simulink model "PassStCalib"  (R2024b)
settings: Solver=FixedStepDiscrete  StartTime=0.0  StopTime=10.0  FixedStep=0.01  RelTol=1e-3
model workspace (MAT data in the model file):
  KeSMSwAcsEntryPassStBkReclnUpwdDnwdPosMax_Val : Simulink.Parameter (value not decoded)
  KeSMSwAcsEntryPassStBkReclnUpwdDnwdPosMin_Val : Simulink.Parameter (value not decoded)
  KeSMSwAcsEntryPassStBkReclnUpwdDnwdPos_Val : Simulink.Parameter (value not decoded)
  KeSMSwAcsEntryPassStFrwdBkwdPosMax_Val : Simulink.Parameter (value not decoded)
  KeSMSwAcsEntryPassStFrwdBkwdPosMin_Val : Simulink.Parameter (value not decoded)
  KeSMSwAcsEntryPassStFrwdBkwdPos_Val : Simulink.Parameter (value not decoded)
  KeSMSwAcsMd56PassStBkReclnUpwdDnwdPosMax_Val : Simulink.Parameter (value not decoded)
  KeSMSwAcsMd56PassStBkReclnUpwdDnwdPosMin_Val : Simulink.Parameter (value not decoded)
  KeSMSwAcsMd56PassStBkReclnUpwdDnwdPos_Val : Simulink.Parameter (value not decoded)
  KeSMSwAcsMd56PassStFrwdBkwdPosMax_Val : Simulink.Parameter (value not decoded)
  KeSMSwAcsMd56PassStFrwdBkwdPosMin_Val : Simulink.Parameter (value not decoded)
  KeSMSwAcsMd56PassStFrwdBkwdPos_Val : Simulink.Parameter (value not decoded)
  KeSMSwRevRMDPassStBkReclnUpwdDnwdPosMax_Val : Simulink.Parameter (value not decoded)
  KeSMSwRevRMDPassStBkReclnUpwdDnwdPosMin_Val : Simulink.Parameter (value not decoded)
  KeSMSwRevRMDPassStBkReclnUpwdDnwdPos_Val : Simulink.Parameter (value not decoded)
  KeSMSwRevRMDPassStFrwdBkwdPosMax_Val : Simulink.Parameter (value not decoded)
  KeSMSwRevRMDPassStFrwdBkwdPosMin_Val : Simulink.Parameter (value not decoded)
  KeSMSwRevRMDPassStFrwdBkwdPos_Val : Simulink.Parameter (value not decoded)
symbols that are objects in the model workspace (value not decoded): KeSMSwAcsEntryPassStBkReclnUpwdDnwdPos_Val, KeSMSwAcsEntryPassStBkReclnUpwdDnwdPosMax_Val, KeSMSwAcsEntryPassStBkReclnUpwdDnwdPosMin_Val, KeSMSwAcsEntryPassStFrwdBkwdPos_Val, KeSMSwAcsEntryPassStFrwdBkwdPosMax_Val, KeSMSwAcsEntryPassStFrwdBkwdPosMin_Val, KeSMSwAcsMd56PassStBkReclnUpwdDnwdPos_Val, KeSMSwAcsMd56PassStBkReclnUpwdDnwdPosMax_Val, KeSMSwAcsMd56PassStBkReclnUpwdDnwdPosMin_Val, KeSMSwAcsMd56PassStFrwdBkwdPos_Val, KeSMSwAcsMd56PassStFrwdBkwdPosMax_Val, KeSMSwAcsMd56PassStFrwdBkwdPosMin_Val, KeSMSwRevRMDPassStBkReclnUpwdDnwdPos_Val, KeSMSwRevRMDPassStBkReclnUpwdDnwdPosMax_Val, KeSMSwRevRMDPassStBkReclnUpwdDnwdPosMin_Val, KeSMSwRevRMDPassStFrwdBkwdPos_Val, KeSMSwRevRMDPassStFrwdBkwdPosMax_Val, KeSMSwRevRMDPassStFrwdBkwdPosMin_Val
undefined symbols (not defined in the file or in its folder): KeSMSuSecRwStVIPFtrstRefAngle_Val, KeSMSw6sAcsEntryPassStFtUpwdDnwdPos_Val, KeSMSw6sAcsEntryPassStFtUpwdDnwdPosMiax_Val, KeSMSw6sAcsEntryPassStFtUpwdDnwdPosMin_Val, KeSMSw6sAcsExtPassStFtUpwdDnwdPos_Val, KeSMSw6sAcsExtPassStFtUpwdDnwdPosMax_Val, KeSMSw6sAcsExtPassStFtUpwdDnwdPosMin_Val, KeSMSw6sRecoveryPassStStFtUpwdDnwdPos_Val, KeSMSw6sRecoveryPassStStFtUpwdDnwdPosMax_Val, KeSMSw6sRecoveryPassStStFtUpwdDnwdPosMin_Val, KeSMSw6SVIPMdPassStBkReclnUpwdDnwdPosPos_Val, KeSMSw6SVIPMdPassStBkReclnUpwdDnwdPosPosMax_Val, KeSMSw6SVIPMdPassStBkReclnUpwdDnwdPosPosMin_Val, KeSMSw6SVIPMdPassStFrwdBkwdPos2_Val, KeSMSw6SVIPMdPassStFrwdBkwdPosMax2_Val, KeSMSw6SVIPMdPassStFrwdBkwdPosMin2_Val, KeSMSw6SVIPMdPassStFrwdBkwdPosPos_Val, KeSMSw6SVIPMdPassStFrwdBkwdPosPosMax_Val, KeSMSw6SVIPMdPassStFrwdBkwdPosPosMin_Val, KeSMSwAcsEntryPassStFtUpwdDnwdPos_Val, KeSMSwAcsEntryPassStFtUpwdDnwdPosMiax_Val, KeSMSwAcsEntryPassStFtUpwdDnwdPosMin_Val, KeSMSwAcsExtPassStFtUpwdDnwdPos_Val, KeSMSwAcsExtPassStFtUpwdDnwdPosMax_Val, KeSMSwAcsExtPassStFtUpwdDnwdPosMin_Val, KeSMSwAcsMd30PassStBkReclnUpwdDnwdPos1_Val, KeSMSwAcsMd30PassStBkReclnUpwdDnwdPos1Max_Val, KeSMSwAcsMd30PassStBkReclnUpwdDnwdPos1Min_Val, KeSMSwAcsMd30PassStBkReclnUpwdDnwdPos_Val, KeSMSwAcsMd30PassStBkReclnUpwdDnwdPosMax_Val, KeSMSwAcsMd30PassStBkReclnUpwdDnwdPosMin_Val, KeSMSwAcsMd30PassStFldUpwdDnwdPos1_Val, KeSMSwAcsMd30PassStFldUpwdDnwdPos1Max_Val, KeSMSwAcsMd30PassStFldUpwdDnwdPos1Min_Val, KeSMSwAcsMd30PassStFldUpwdDnwdPos_Val, KeSMSwAcsMd30PassStFldUpwdDnwdPosMax_Val, KeSMSwAcsMd30PassStFldUpwdDnwdPosMin_Val, KeSMSwAcsMd30PassStFrwdBkwdPos1_Val, KeSMSwAcsMd30PassStFrwdBkwdPos1Max_Val, KeSMSwAcsMd30PassStFrwdBkwdPos1Min_Val, KeSMSwAcsMd30PassStFrwdBkwdPos_Val, KeSMSwAcsMd30PassStFrwdBkwdPosMax_Val, KeSMSwAcsMd30PassStFrwdBkwdPosMin_Val, KeSMSwAcsMd31PassStBkReclnUpwdDnwdPos1_Val, KeSMSwAcsMd31PassStBkReclnUpwdDnwdPos1Max_Val, KeSMSwAcsMd31PassStBkReclnUpwdDnwdPos1Min_Val, KeSMSwAcsMd31PassStBkReclnUpwdDnwdPos_Val, KeSMSwAcsMd31PassStBkReclnUpwdDnwdPosMax_Val, KeSMSwAcsMd31PassStBkReclnUpwdDnwdPosMin_Val, KeSMSwAcsMd31PassStFldUpwdDnwdPos_Val, KeSMSwAcsMd31PassStFldUpwdDnwdPosMax_Val, KeSMSwAcsMd31PassStFldUpwdDnwdPosMin_Val, KeSMSwAcsMd31PassStFrwdBkwdPos1_Val, KeSMSwAcsMd31PassStFrwdBkwdPos1Max_Val, KeSMSwAcsMd31PassStFrwdBkwdPos1Min_Val, KeSMSwAcsMd31PassStFrwdBkwdPos_Val, KeSMSwAcsMd31PassStFrwdBkwdPosMax_Val, KeSMSwAcsMd31PassStFrwdBkwdPosMin_Val, KeSMSwAcsMd57PassStBkReclnUpwdDnwdPosPos_Val, KeSMSwAcsMd57PassStBkReclnUpwdDnwdPosPosMax_Val ... (+34)
libraries: TrgtPosSelcLib x20
(part 3 of 3)

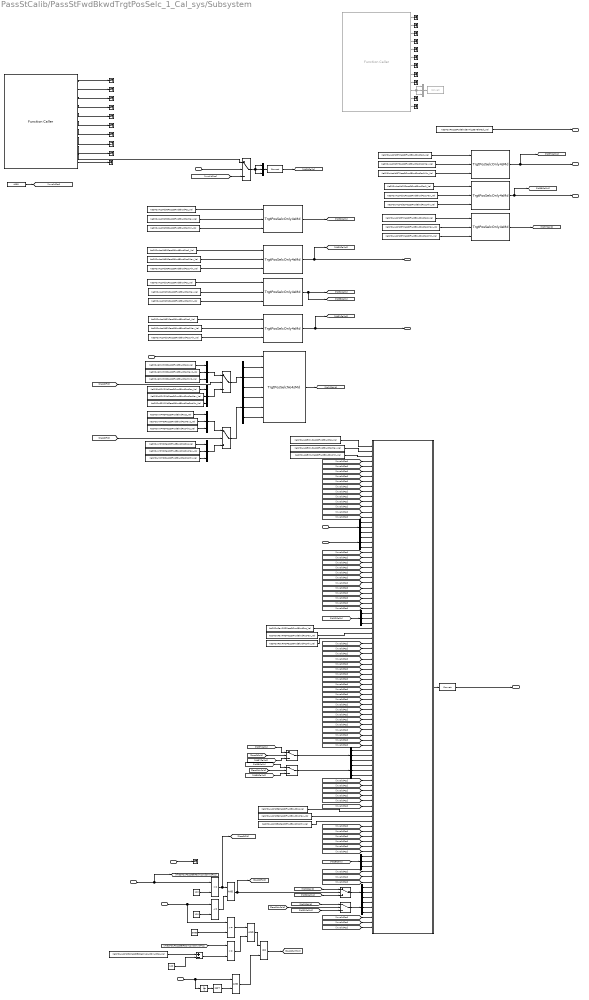
== system PassStCalib/PassStFwdBkwdTrgtPosSelc_1_Cal_sys/Subsystem ==
  note: 副驾折叠判断条件更改
  note: Delete block
  IfVeSMSbSecRwRtStCshnFrntUpwdDnwdMovConfig_Val_read : Inport
  Md30BkStgDone_Val_read : Inport  Port=2
  Md31BkStgDone_Val_read : Inport  Port=3
  StNumFlg_Is6s_read : Inport  Port=4
  IfVeSMSuPassStBkReclnUpwdDnwdPos_Val_read : Inport  Port=5
  IfVeSMSuPassStFldUpwdDnwdPos_Val_read : Inport  Port=6
  Md61PassStFwdBkwdTrgtPosCalib_TrgtPosArray_read : Inport  Port=7
  Md62PassStFwdBkwdTrgtPosCalib_TrgtPosArray_read : Inport  Port=8
  Constant : Constant  Value=4095  OutDataTypeStr=uint16
  Constant1 : Constant  Value=120  OutDataTypeStr=uint16
  Constant2 : Constant  Value=120  OutDataTypeStr=uint16
  Constant3 : Constant  Value=3880  OutDataTypeStr=uint16
  Constant4 : Constant  Value=120  OutDataTypeStr=uint16
  Data Type Conversion1 : DataTypeConversion  Commented=on  SaturateOnIntegerOverflow=off  RndMeth=Floor
  Data Type Conversion2 : DataTypeConversion  SaturateOnIntegerOverflow=off  RndMeth=Floor
  Data Type Conversion3 : DataTypeConversion  SaturateOnIntegerOverflow=off  RndMeth=Floor
  Demux{,1..9} (10 alike) : Demux  Outputs=3
  Logical Operator : Logic  AllPortsSameDT=off  OutDataTypeStr=boolean
  Logical Operator2 : Logic  Operator=OR  AllPortsSameDT=off  OutDataTypeStr=boolean
  Logical Operator3 : Logic  AllPortsSameDT=off  OutDataTypeStr=boolean
  Logical Operator4 : Logic  AllPortsSameDT=off  OutDataTypeStr=boolean
  Logical Operator5 : Logic  Operator=NOT  AllPortsSameDT=off  OutDataTypeStr=boolean
  Md58TrgtPos_Get : FunctionCaller  Commented=on  FunctionPrototype=[SecRwRtStBkReclnTrgtPos,SecRwRtStZeroTrgtPos,SecRwRtStLgrstUpwdDnwdTrgtPos,SecRwRtStLgrstInwdOtwdTrgtPos,ThdRwLtStBkReclnTrgtPos,ThdRwLtStFwdBkwdTrgtPos,ThdRwRtStBkReclnTrgtPos,ThdRwRtStFwdBkwdTrgtPos,PassStBkReclnTrgtPos,PassStFwdBkwdTrgtPos,SecRwRtStFwdBkwdTrgtPos,PassStFldTrgtPos] = Md58TrgtPos_Get()  InputArgumentSpecifications=<Enter example>  OutputArgumentSpecifications=uint16(1), uint16(1), uint16(1), uint16(1), uint16(1), uint16(1), uint16(1), uint16(1), uint16(1), uint16(1), uint16(1), uint16(1)
  Mux{,2..5} (5 alike) : Mux  Inputs=3
  Mux1 : Mux  Commented=on  Inputs=3
  PA_KeSMSw6SVIPMdPassStFrwdBkwdPos2_Val : Constant  Value=KeSMSw6SVIPMdPassStFrwdBkwdPos2_Val
  PA_KeSMSw6SVIPMdPassStFrwdBkwdPosMax2_Val : Constant  Value=KeSMSw6SVIPMdPassStFrwdBkwdPosMax2_Val
  PA_KeSMSw6SVIPMdPassStFrwdBkwdPosMin2_Val : Constant  Value=KeSMSw6SVIPMdPassStFrwdBkwdPosMin2_Val
  PA_KeSMSw6SVIPMdPassStFrwdBkwdPosPosMax_Val : Constant  Value=KeSMSw6SVIPMdPassStFrwdBkwdPosPosMax_Val
  PA_KeSMSw6SVIPMdPassStFrwdBkwdPosPosMin_Val : Constant  Value=KeSMSw6SVIPMdPassStFrwdBkwdPosPosMin_Val
  PA_KeSMSw6SVIPMdPassStFrwdBkwdPosPos_Val : Constant  Value=KeSMSw6SVIPMdPassStFrwdBkwdPosPos_Val
  PA_KeSMSwAcsEntryPassStFrwdBkwdPosMax_Val : Constant  Value=KeSMSwAcsEntryPassStFrwdBkwdPosMax_Val
  PA_KeSMSwAcsEntryPassStFrwdBkwdPosMin_Val : Constant  Value=KeSMSwAcsEntryPassStFrwdBkwdPosMin_Val
  PA_KeSMSwAcsEntryPassStFrwdBkwdPos_Val : Constant  Value=KeSMSwAcsEntryPassStFrwdBkwdPos_Val
  PA_KeSMSwAcsMd30PassStFrwdBkwdPos1Max_Val : Constant  Value=KeSMSwAcsMd30PassStFrwdBkwdPos1Max_Val
  PA_KeSMSwAcsMd30PassStFrwdBkwdPos1Min_Val : Constant  Value=KeSMSwAcsMd30PassStFrwdBkwdPos1Min_Val
  PA_KeSMSwAcsMd30PassStFrwdBkwdPos1_Val : Constant  Value=KeSMSwAcsMd30PassStFrwdBkwdPos1_Val
  PA_KeSMSwAcsMd30PassStFrwdBkwdPosMax_Val : Constant  Value=KeSMSwAcsMd30PassStFrwdBkwdPosMax_Val
  PA_KeSMSwAcsMd30PassStFrwdBkwdPosMin_Val : Constant  Value=KeSMSwAcsMd30PassStFrwdBkwdPosMin_Val
  PA_KeSMSwAcsMd30PassStFrwdBkwdPos_Val : Constant  Value=KeSMSwAcsMd30PassStFrwdBkwdPos_Val
  PA_KeSMSwAcsMd31PassStBkReclnUpwdDnwdPos_Val : Constant  Value=KeSMSwAcsMd31PassStBkReclnUpwdDnwdPos_Val
  PA_KeSMSwAcsMd31PassStFrwdBkwdPos1Max_Val : Constant  Value=KeSMSwAcsMd31PassStFrwdBkwdPos1Max_Val
  PA_KeSMSwAcsMd31PassStFrwdBkwdPos1Max_Val1 : Constant  Value=KeSMSwAcsMd31PassStFrwdBkwdPos1Max_Val
  PA_KeSMSwAcsMd31PassStFrwdBkwdPos1Min_Val : Constant  Value=KeSMSwAcsMd31PassStFrwdBkwdPos1Min_Val
  PA_KeSMSwAcsMd31PassStFrwdBkwdPos1Min_Val1 : Constant  Value=KeSMSwAcsMd31PassStFrwdBkwdPos1Min_Val
  PA_KeSMSwAcsMd31PassStFrwdBkwdPos1_Val : Constant  Value=KeSMSwAcsMd31PassStFrwdBkwdPos1_Val
  PA_KeSMSwAcsMd31PassStFrwdBkwdPos1_Val1 : Constant  Value=KeSMSwAcsMd31PassStFrwdBkwdPos1_Val
  PA_KeSMSwAcsMd31PassStFrwdBkwdPosMax_Val : Constant  Value=KeSMSwAcsMd31PassStFrwdBkwdPosMax_Val
  PA_KeSMSwAcsMd31PassStFrwdBkwdPosMin_Val : Constant  Value=KeSMSwAcsMd31PassStFrwdBkwdPosMin_Val
  PA_KeSMSwAcsMd31PassStFrwdBkwdPos_Val : Constant  Value=KeSMSwAcsMd31PassStFrwdBkwdPos_Val
  PA_KeSMSwAcsMd56PassStFrwdBkwdPosMax_Val : Constant  Value=KeSMSwAcsMd56PassStFrwdBkwdPosMax_Val
  PA_KeSMSwAcsMd56PassStFrwdBkwdPosMin_Val : Constant  Value=KeSMSwAcsMd56PassStFrwdBkwdPosMin_Val
  PA_KeSMSwAcsMd56PassStFrwdBkwdPos_Val : Constant  Value=KeSMSwAcsMd56PassStFrwdBkwdPos_Val
  PA_KeSMSwAcsMd57PassStFrwdBkwdPosPos1Max_Val : Constant  Value=KeSMSwAcsMd57PassStFrwdBkwdPosPos1Max_Val
  PA_KeSMSwAcsMd57PassStFrwdBkwdPosPos1Min_Val : Constant  Value=KeSMSwAcsMd57PassStFrwdBkwdPosPos1Min_Val
  PA_KeSMSwAcsMd57PassStFrwdBkwdPosPos1_Val : Constant  Value=KeSMSwAcsMd57PassStFrwdBkwdPosPos1_Val
  PA_KeSMSwAcsMd57PassStFrwdBkwdPosPos2Max_Val : Constant  Value=KeSMSwAcsMd57PassStFrwdBkwdPosPos2Max_Val
  PA_KeSMSwAcsMd57PassStFrwdBkwdPosPos2Min_Val : Constant  Value=KeSMSwAcsMd57PassStFrwdBkwdPosPos2Min_Val
  PA_KeSMSwAcsMd57PassStFrwdBkwdPosPos2_Val : Constant  Value=KeSMSwAcsMd57PassStFrwdBkwdPosPos2_Val
  PA_KeSMSwPassStFwdBkwdEnTrig557BitMask_Val : Constant  Value=KeSMSwPassStFwdBkwdEnTrig557BitMask_Val
  PA_KeSMSwRevRMDPassStFrwdBkwdPosMax_Val : Constant  Value=KeSMSwRevRMDPassStFrwdBkwdPosMax_Val
  PA_KeSMSwRevRMDPassStFrwdBkwdPosMin_Val : Constant  Value=KeSMSwRevRMDPassStFrwdBkwdPosMin_Val
  PA_KeSMSwRevRMDPassStFrwdBkwdPos_Val : Constant  Value=KeSMSwRevRMDPassStFrwdBkwdPos_Val
  PA_KeSMSwVIPMDPassStFrwdBkwdPos2_Val : Constant  Value=KeSMSwVIPMDPassStFrwdBkwdPos2_Val
  PA_KeSMSwVIPMDPassStFrwdBkwdPosMax2_Val : Constant  Value=KeSMSwVIPMDPassStFrwdBkwdPosMax2_Val
  PA_KeSMSwVIPMDPassStFrwdBkwdPosMin2_Val : Constant  Value=KeSMSwVIPMDPassStFrwdBkwdPosMin2_Val
  PA_KeSMSwVIPMDPassStFrwdBkwdPosPosMax_Val : Constant  Value=KeSMSwVIPMDPassStFrwdBkwdPosPosMax_Val
  PA_KeSMSwVIPMDPassStFrwdBkwdPosPosMin_Val : Constant  Value=KeSMSwVIPMDPassStFrwdBkwdPosPosMin_Val
  PA_KeSMSwVIPMDPassStFrwdBkwdPosPos_Val : Constant  Value=KeSMSwVIPMDPassStFrwdBkwdPosPos_Val
  Relational Operator : RelationalOperator  Operator=<=  OutDataTypeStr=boolean  RndMeth=Simplest  InputSameDT=off
  Relational Operator1 : RelationalOperator  Operator=<=  OutDataTypeStr=boolean  RndMeth=Simplest  InputSameDT=off
  Relational Operator2 : RelationalOperator  OutDataTypeStr=boolean  RndMeth=Simplest  InputSameDT=off
  Relational Operator3 : RelationalOperator  OutDataTypeStr=boolean  RndMeth=Simplest  InputSameDT=off
  Subsystem : Subsystem
  Subtract : Sum  Inputs=+-  OutDataTypeStr=uint16  AccumDataTypeStr=uint16
  Switch{,1..6} (7 alike) : Switch  Criteria=u2 > Threshold  SaturateOnIntegerOverflow=off  InputSameDT=off
  Terminator{,1..9} (10 alike) : Terminator
  Terminator_{10..21} (12 alike) : Terminator
  TrgtPosSelcNo4sMd : TrgtPosSelcLib/TrgtPosSelcNo4sMd  SystemSampleTime=-1  VariantActivationTime=update diagram  AllowFlexibleInterface=on  Latency=0  AutoFrameSizeCalculation=off
  TrgtPosSelcOnly4sMd{,1..6} (7 alike) : TrgtPosSelcLib/TrgtPosSelcOnly4sMd  SystemSampleTime=-1  VariantActivationTime=update diagram  AllowFlexibleInterface=on  Latency=0  AutoFrameSizeCalculation=off
  Unit Delay : UnitDelay  SampleTime=-1  HasFrameUpgradeWarning=on
  VIPRExit557TrgtPos_Get : FunctionCaller  FunctionPrototype=[SecRwRtStBkReclnTrgtPos,SecRwRtStZeroTrgtPos,SecRwRtStLgrstUpwdDnwdTrgtPos,SecRwRtStLgrstInwdOtwdTrgtPos,ThdRwLtStBkReclnTrgtPos,ThdRwLtStFwdBkwdTrgtPos,ThdRwRtStBkReclnTrgtPos,ThdRwRtStFwdBkwdTrgtPos,PassStBkReclnTrgtPos,PassStFwdBkwdTrgtPos,SecRwRtStFwdBkwdTrgtPos] = VIPRExit557TrgtPos_Get()  InputArgumentSpecifications=<Enter example>  OutputArgumentSpecifications=uint16(1), uint16(1), uint16(1), uint16(1), uint16(1), uint16(1), uint16(1), uint16(1), uint16(1), uint16(1), uint16(1)
  Md30PassStFwdBkwdTrgtPosCalib1_TrgtPosArray_write : Outport  VectorParamsAs1DForOutWhenUnconnected=off
      settings: EnsureOutportIsVirtual=on
  Md31PassStFwdBkwdTrgtPosCalib1_TrgtPosArray_write : Outport  Port=2  VectorParamsAs1DForOutWhenUnconnected=off
      settings: EnsureOutportIsVirtual=on
  PassStFwdBkwdTrgtPosCalibArray32_TrgtPosArray32_write : Outport  Port=3  VectorParamsAs1DForOutWhenUnconnected=off
      settings: EnsureOutportIsVirtual=on
  Md57PassStFwdBkwdTrgtPosCalib1_TrgtPosArray_write : Outport  Port=4  VectorParamsAs1DForOutWhenUnconnected=off
      settings: EnsureOutportIsVirtual=on
  Md58PassStFwdBkwdTrgtPosCalib1_TrgtPosArray_write : Outport  Port=5  VectorParamsAs1DForOutWhenUnconnected=off
      settings: EnsureOutportIsVirtual=on
  PassStFwdBkwdStEnTrigBitMask_Val_write : Outport  Port=6  VectorParamsAs1DForOutWhenUnconnected=off
      settings: EnsureOutportIsVirtual=on
  wires:
  TrgtPosSelcOnly4sMd/1 -> [Md30Calib]
  TrgtPosSelcOnly4sMd1/1 -> [Md30Calib1], Md30PassStFwdBkwdTrgtPosCalib1_TrgtPosArray_write/1
  TrgtPosSelcOnly4sMd2/1 -> [Md58Calib], [Md31Calib]
  TrgtPosSelcOnly4sMd3/1 -> [Md31Calib1], Md31PassStFwdBkwdTrgtPosCalib1_TrgtPosArray_write/1
  PA_KeSMSwAcsMd30PassStFrwdBkwdPosMin_Val/1 -> TrgtPosSelcOnly4sMd/3
  PA_KeSMSwAcsMd30PassStFrwdBkwdPosMax_Val/1 -> TrgtPosSelcOnly4sMd/2
  PA_KeSMSwAcsMd30PassStFrwdBkwdPos_Val/1 -> TrgtPosSelcOnly4sMd/1
  PA_KeSMSwAcsMd30PassStFrwdBkwdPos1Max_Val/1 -> TrgtPosSelcOnly4sMd1/2
  PA_KeSMSwAcsMd30PassStFrwdBkwdPos1Min_Val/1 -> TrgtPosSelcOnly4sMd1/3
  PA_KeSMSwAcsMd30PassStFrwdBkwdPos1_Val/1 -> TrgtPosSelcOnly4sMd1/1
  PA_KeSMSwAcsMd31PassStFrwdBkwdPosMax_Val/1 -> TrgtPosSelcOnly4sMd2/2
  PA_KeSMSwAcsMd31PassStFrwdBkwdPosMin_Val/1 -> TrgtPosSelcOnly4sMd2/3
  PA_KeSMSwAcsMd31PassStFrwdBkwdPos_Val/1 -> TrgtPosSelcOnly4sMd2/1
  PA_KeSMSwAcsMd31PassStFrwdBkwdPos1_Val/1 -> TrgtPosSelcOnly4sMd3/1
  PA_KeSMSwAcsMd31PassStFrwdBkwdPos1Max_Val/1 -> TrgtPosSelcOnly4sMd3/2
  PA_KeSMSwAcsMd31PassStFrwdBkwdPos1Min_Val/1 -> TrgtPosSelcOnly4sMd3/3
  Data Type Conversion2/1 -> [Md28Calib]
  Switch/1 -> Mux/3, Mux/1, Mux/2
  VIPRExit557TrgtPos_Get/10 -> Switch/1
  Mux/1 -> Data Type Conversion2/1
  IfVeSMSbSecRwRtStCshnFrntUpwdDnwdMovConfig_Val_read/1 -> Switch/2
  [invalidPos] -> Switch/3
  Constant/1 -> [invalidPos]
  StNumFlg_Is6s_read/1 -> TrgtPosSelcNo4sMd/1
  TrgtPosSelcNo4sMd/1 -> [Md12Calib]
  Demux4/1 -> Subsystem/61(Md21Pos)
  Demux5/2 -> Subsystem/65(Md22PosMax)
  Demux5/1 -> Subsystem/64(Md22Pos)
  [invalidPos] -> Subsystem/56(Md19PosMax)
  PA_KeSMSwRevRMDPassStFrwdBkwdPosMax_Val/1 -> Subsystem/38(Md13PosMax)
  [invalidPos] -> Subsystem/69(Md23PosMin)
  [invalidPos] -> Subsystem/46(Md16Pos)
  [invalidPos] -> Subsystem/54(Md18PosMin)
  Demux/1 -> Subsystem/34(Md12Pos)
  [invalidPos] -> Subsystem/52(Md18Pos)
  [invalidPos] -> Subsystem/58(Md20Pos)
  [invalidPos] -> Subsystem/32(Md11PosMax)
  Demux/2 -> Subsystem/35(Md12PosMax)
  [invalidPos] -> Subsystem/55(Md19Pos)
  [invalidPos] -> Subsystem/5(Md2PosMax)
  [invalidPos] -> Subsystem/26(Md9PosMax)
  [invalidPos] -> Subsystem/31(Md11Pos)
  [invalidPos] -> Subsystem/28(Md10Pos)
  PA_KeSMSwRevRMDPassStFrwdBkwdPos_Val/1 -> Subsystem/37(Md13Pos)
  [invalidPos] -> Subsystem/25(Md9Pos)
  Demux8/3 -> Subsystem/21(Md7PosMin)
  [invalidPos] -> Subsystem/43(Md15Pos)
  Demux8/2 -> Subsystem/20(Md7PosMax)
  PA_KeSMSwAcsEntryPassStFrwdBkwdPosMin_Val/1 -> Subsystem/3(Md1Min)
  [invalidPos] -> Subsystem/30(Md10PosMin)
  Data Type Conversion3/1 -> PassStFwdBkwdTrgtPosCalibArray32_TrgtPosArray32_write/1
  [invalidPos] -> Subsystem/68(Md23PosMax)
  [invalidPos] -> Subsystem/15(Md5PosMin)
  Demux3/2 -> Subsystem/92(Md31PosMax)
  [invalidPos] -> Subsystem/50(Md17PosMax)
  [invalidPos] -> Subsystem/44(Md15PosMax)
  [invalidPos] -> Subsystem/70(Md24Pos)
  [invalidPos] -> Subsystem/79(Md27Pos)
  Demux2/3 -> Subsystem/90(Md30PosMin)
  [invalidPos] -> Subsystem/81(Md27PosMin)
  Demux3/1 -> Subsystem/91(Md31Pos)
  Demux2/1 -> Subsystem/88(Md30Pos)
  Demux5/3 -> Subsystem/66(Md22PosMin)
  [invalidPos] -> Subsystem/22(Md8Pos)
  [invalidPos] -> Subsystem/86(Md29PosMax)
  Demux2/2 -> Subsystem/89(Md30PosMax)
  Demux1/3 -> Subsystem/84(Md28PosMin)
  [invalidPos] -> Subsystem/85(Md29Pos)
  Demux1/1 -> Subsystem/82(Md28Pos)
  PA_KeSMSwRevRMDPassStFrwdBkwdPosMin_Val/1 -> Subsystem/39(Md13PosMin)
  Demux/3 -> Subsystem/36(Md12PosMin)
  [invalidPos] -> Subsystem/13(Md5Pos)
  PA_KeSMSwAcsMd56PassStFrwdBkwdPos_Val/1 -> Subsystem/73(Md25Pos)
  [invalidPos] -> Subsystem/29(Md10PosMax)
  [invalidPos] -> Subsystem/94(Md32Pos)
  Demux9/3 -> Subsystem/18(Md6PosMin)
  PA_KeSMSwAcsEntryPassStFrwdBkwdPosMax_Val/1 -> Subsystem/2(Md1Max)
  Demux1/2 -> Subsystem/83(Md28PosMax)
  [Md12Calib] -> Demux/1
  [invalidPos] -> Subsystem/95(Md32PosMax)
  [invalidPos] -> Subsystem/51(Md17PosMin)
  Demux3/3 -> Subsystem/93(Md31PosMin)
  [invalidPos] -> Subsystem/57(Md19PosMin)
  [invalidPos] -> Subsystem/45(Md15PosMin)
  Demux4/3 -> Subsystem/63(Md21PosMin)
  PA_KeSMSwAcsMd56PassStFrwdBkwdPosMax_Val/1 -> Subsystem/74(Md25PosMax)
  [invalidPos] -> Subsystem/41(Md14PosMax)
  [invalidPos] -> Subsystem/71(Md24PosMax)
  [Md28Calib] -> Demux1/1
  [invalidPos] -> Subsystem/14(Md5PosMax)
  [invalidPos] -> Subsystem/76(Md26Pos)
  [invalidPos] -> Subsystem/49(Md17Pos)
  [invalidPos] -> Subsystem/27(Md9PosMin)
  [invalidPos] -> Subsystem/87(Md29PosMin)
  [invalidPos] -> Subsystem/40(Md14Pos)
  [invalidPos] -> Subsystem/24(Md8PosMin)
  [invalidPos] -> Subsystem/59(Md20PosMax)
  [invalidPos] -> Subsystem/47(Md16PosMax)
  [invalidPos] -> Subsystem/96(Md32PosMin)
  [invalidPos] -> Subsystem/80(Md27PosMax)
  [invalidPos] -> Subsystem/48(Md16PosMin)
  [invalidPos] -> Subsystem/42(Md14PosMin)
  PA_KeSMSwAcsMd56PassStFrwdBkwdPosMin_Val/1 -> Subsystem/75(Md25PosMin)
  Demux8/1 -> Subsystem/19(Md7Pos)
  [invalidPos] -> Subsystem/53(Md18PosMax)
  PA_KeSMSwAcsEntryPassStFrwdBkwdPos_Val/1 -> Subsystem/1(Md1Pos)
  [invalidPos] -> Subsystem/7(Md3Pos)
  Demux4/2 -> Subsystem/62(Md21PosMax)
  [invalidPos] -> Subsystem/33(Md11PosMin)
  [invalidPos] -> Subsystem/4(Md2Pos)
  [invalidPos] -> Subsystem/72(Md24PosMin)
  [invalidPos] -> Subsystem/8(Md3PosMax)
  Demux9/1 -> Subsystem/16(Md6Pos)
  [invalidPos] -> Subsystem/10(Md4Pos)
  [invalidPos] -> Subsystem/6(Md2PosMin)
  [invalidPos] -> Subsystem/9(Md3PosMin)
  [invalidPos] -> Subsystem/67(Md23Pos)
  [invalidPos] -> Subsystem/23(Md8PosMax)
  [invalidPos] -> Subsystem/60(Md20PosMin)
  [invalidPos] -> Subsystem/78(Md26PosMin)
  [invalidPos] -> Subsystem/11(Md4PosMax)
  Subsystem/1(CalibArray32) -> Data Type Conversion3/1
  [invalidPos] -> Subsystem/12(Md4PosMin)
  [invalidPos] -> Subsystem/77(Md26PosMax)
  Demux9/2 -> Subsystem/17(Md6PosMax)
  Switch1/1 -> Demux2/1
  [Md30Calib] -> Switch1/1
  [Md30Calib1] -> Switch1/3
  Switch2/1 -> Demux3/1
  VIPRExit557TrgtPos_Get/1 -> Terminator/1
  VIPRExit557TrgtPos_Get/2 -> Terminator1/1
  VIPRExit557TrgtPos_Get/3 -> Terminator2/1
  VIPRExit557TrgtPos_Get/4 -> Terminator3/1
  VIPRExit557TrgtPos_Get/5 -> Terminator4/1
  VIPRExit557TrgtPos_Get/6 -> Terminator5/1
  VIPRExit557TrgtPos_Get/7 -> Terminator6/1
  VIPRExit557TrgtPos_Get/8 -> Terminator7/1
  VIPRExit557TrgtPos_Get/9 -> Terminator8/1
  VIPRExit557TrgtPos_Get/11 -> Terminator_10/1
  IfVeSMSuPassStBkReclnUpwdDnwdPos_Val_read/1 -> [IfVeSMSuPassStBkReclnUpwdDnwdPos], Relational Operator/1
  IfVeSMSuPassStFldUpwdDnwdPos_Val_read/1 -> Relational Operator2/1, Relational Operator1/1
  Constant1/1 -> Relational Operator/2
  Constant2/1 -> Relational Operator1/2
  Relational Operator/1 -> [PassStFld], Logical Operator/1
  Relational Operator1/1 -> Logical Operator/2
  Constant3/1 -> Relational Operator2/2
  Logical Operator/1 -> Switch1/2, [PassStFold]
  Relational Operator2/1 -> Logical Operator3/1
  PA_KeSMSwPassStFwdBkwdEnTrig557BitMask_Val/1 -> PassStFwdBkwdStEnTrigBitMask_Val_write/1
  PA_KeSMSwAcsMd57PassStFrwdBkwdPosPos1Max_Val/1 -> TrgtPosSelcOnly4sMd4/2
  PA_KeSMSwAcsMd57PassStFrwdBkwdPosPos1Min_Val/1 -> TrgtPosSelcOnly4sMd4/3
  PA_KeSMSwAcsMd57PassStFrwdBkwdPosPos1_Val/1 -> TrgtPosSelcOnly4sMd4/1
  TrgtPosSelcOnly4sMd4/1 -> [Md57Calib1], Md57PassStFwdBkwdTrgtPosCalib1_TrgtPosArray_write/1
  PA_KeSMSwAcsMd31PassStFrwdBkwdPos1Max_Val1/1 -> TrgtPosSelcOnly4sMd5/2
  PA_KeSMSwAcsMd31PassStFrwdBkwdPos1Min_Val1/1 -> TrgtPosSelcOnly4sMd5/3
  PA_KeSMSwAcsMd31PassStFrwdBkwdPos1_Val1/1 -> TrgtPosSelcOnly4sMd5/1
  TrgtPosSelcOnly4sMd5/1 -> [Md58Calib1], Md58PassStFwdBkwdTrgtPosCalib1_TrgtPosArray_write/1
  PA_KeSMSwAcsMd57PassStFrwdBkwdPosPos2Max_Val/1 -> TrgtPosSelcOnly4sMd6/2
  PA_KeSMSwAcsMd57PassStFrwdBkwdPosPos2Min_Val/1 -> TrgtPosSelcOnly4sMd6/3
  PA_KeSMSwAcsMd57PassStFrwdBkwdPosPos2_Val/1 -> TrgtPosSelcOnly4sMd6/1
  TrgtPosSelcOnly4sMd6/1 -> [Md57Calib]
  Mux1/1 -> Data Type Conversion1/1
  Md58TrgtPos_Get/10 -> Mux1/2, Mux1/1, Mux1/3
  [PassStFold] -> Switch3/2
  [PassStUnFold] -> Switch4/2
  [Md57Calib] -> Switch3/1
  Switch3/1 -> Demux4/1
  [Md58Calib] -> Switch4/1
  Switch4/1 -> Demux5/1
  [Md57Calib1] -> Switch3/3
  [Md58Calib1] -> Switch4/3
  Md58TrgtPos_Get/1 -> Terminator_11/1
  Md58TrgtPos_Get/2 -> Terminator_12/1
  Md58TrgtPos_Get/3 -> Terminator_13/1
  Md58TrgtPos_Get/4 -> Terminator_14/1
  Md58TrgtPos_Get/5 -> Terminator_15/1
  Md58TrgtPos_Get/6 -> Terminator_16/1
  Md58TrgtPos_Get/7 -> Terminator_17/1
  Md58TrgtPos_Get/8 -> Terminator_18/1
  Md58TrgtPos_Get/9 -> Terminator_19/1
  Md58TrgtPos_Get/11 -> Terminator_20/1
  Md58TrgtPos_Get/12 -> Terminator_21/1
  [IfVeSMSuPassStBkReclnUpwdDnwdPos] -> Relational Operator3/1
  Relational Operator3/1 -> Logical Operator3/2
  [Md31Calib1] -> Switch2/3
  [Md31Calib] -> Switch2/1
  Md31BkStgDone_Val_read/1 -> Unit Delay/1, Logical Operator4/1
  Logical Operator2/1 -> [PassStUnFold]
  [PassStUnFold] -> Switch2/2
  Logical Operator3/1 -> Logical Operator2/1
  Unit Delay/1 -> Logical Operator5/1
  Logical Operator5/1 -> Logical Operator4/2
  Logical Operator4/1 -> Logical Operator2/2
  Subtract/1 -> Relational Operator3/2
  PA_KeSMSwAcsMd31PassStBkReclnUpwdDnwdPos_Val/1 -> Subtract/1
  Constant4/1 -> Subtract/2
  [PassStFld] -> Switch5/2
  Demux6/2 -> TrgtPosSelcNo4sMd/3
  Demux6/1 -> TrgtPosSelcNo4sMd/2
  Demux6/3 -> TrgtPosSelcNo4sMd/4
  Switch5/1 -> Demux6/1
  Mux2/1 -> Switch5/1
  PA_KeSMSw6SVIPMdPassStFrwdBkwdPos2_Val/1 -> Mux2/1
  PA_KeSMSw6SVIPMdPassStFrwdBkwdPosMax2_Val/1 -> Mux2/2
  PA_KeSMSw6SVIPMdPassStFrwdBkwdPosMin2_Val/1 -> Mux2/3
  Mux3/1 -> Switch5/3
  PA_KeSMSw6SVIPMdPassStFrwdBkwdPosPos_Val/1 -> Mux3/1
  PA_KeSMSw6SVIPMdPassStFrwdBkwdPosPosMax_Val/1 -> Mux3/2
  PA_KeSMSw6SVIPMdPassStFrwdBkwdPosPosMin_Val/1 -> Mux3/3
  Demux7/3 -> TrgtPosSelcNo4sMd/7
  Demux7/1 -> TrgtPosSelcNo4sMd/5
  Demux7/2 -> TrgtPosSelcNo4sMd/6
  Switch6/1 -> Demux7/1
  Mux4/1 -> Switch6/1
  PA_KeSMSwVIPMDPassStFrwdBkwdPos2_Val/1 -> Mux4/1
  PA_KeSMSwVIPMDPassStFrwdBkwdPosMax2_Val/1 -> Mux4/2
  PA_KeSMSwVIPMDPassStFrwdBkwdPosMin2_Val/1 -> Mux4/3
  Mux5/1 -> Switch6/3
  PA_KeSMSwVIPMDPassStFrwdBkwdPosPosMin_Val/1 -> Mux5/3
  PA_KeSMSwVIPMDPassStFrwdBkwdPosPosMax_Val/1 -> Mux5/2
  PA_KeSMSwVIPMDPassStFrwdBkwdPosPos_Val/1 -> Mux5/1
  [PassStFld] -> Switch6/2
  Md61PassStFwdBkwdTrgtPosCalib_TrgtPosArray_read/1 -> Demux9/1
  Md62PassStFwdBkwdTrgtPosCalib_TrgtPosArray_read/1 -> Demux8/1
  Md30BkStgDone_Val_read/1 -> Terminator9/1

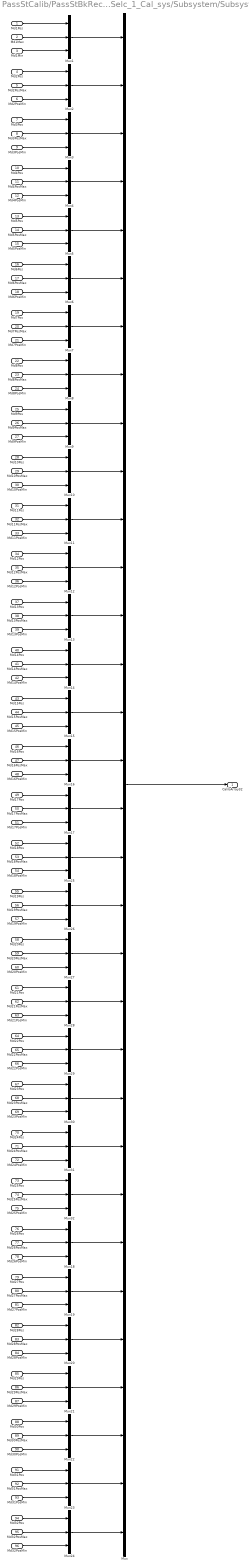
== system PassStCalib/PassStBkReclnTrgtPosSelc_1_Cal_sys/Subsystem/Subsystem ==
  Md1Pos : Inport
  Md1Max : Inport  Port=2
  Md1Min : Inport  Port=3
  Md2Pos : Inport  Port=4
  Md2PosMax : Inport  Port=5
  Md2PosMin : Inport  Port=6
  Md3Pos : Inport  Port=7
  Md3PosMax : Inport  Port=8
  Md3PosMin : Inport  Port=9
  Md4Pos : Inport  Port=10
  Md4PosMax : Inport  Port=11
  Md4PosMin : Inport  Port=12
  Md5Pos : Inport  Port=13
  Md5PosMax : Inport  Port=14
  Md5PosMin : Inport  Port=15
  Md6Pos : Inport  Port=16
  Md6PosMax : Inport  Port=17
  Md6PosMin : Inport  Port=18
  Md7Pos : Inport  Port=19
  Md7PosMax : Inport  Port=20
  Md7PosMin : Inport  Port=21
  Md8Pos : Inport  Port=22
  Md8PosMax : Inport  Port=23
  Md8PosMin : Inport  Port=24
  Md9Pos : Inport  Port=25
  Md9PosMax : Inport  Port=26
  Md9PosMin : Inport  Port=27
  Md10Pos : Inport  Port=28
  Md10PosMax : Inport  Port=29
  Md10PosMin : Inport  Port=30
  Md11Pos : Inport  Port=31
  Md11PosMax : Inport  Port=32
  Md11PosMin : Inport  Port=33
  Md12Pos : Inport  Port=34
  Md12PosMax : Inport  Port=35
  Md12PosMin : Inport  Port=36
  Md13Pos : Inport  Port=37
  Md13PosMax : Inport  Port=38
  Md13PosMin : Inport  Port=39
  Md14Pos : Inport  Port=40
  Md14PosMax : Inport  Port=41
  Md14PosMin : Inport  Port=42
  Md15Pos : Inport  Port=43
  Md15PosMax : Inport  Port=44
  Md15PosMin : Inport  Port=45
  Md16Pos : Inport  Port=46
  Md16PosMax : Inport  Port=47
  Md16PosMin : Inport  Port=48
  Md17Pos : Inport  Port=49
  Md17PosMax : Inport  Port=50
  Md17PosMin : Inport  Port=51
  Md18Pos : Inport  Port=52
  Md18PosMax : Inport  Port=53
  Md18PosMin : Inport  Port=54
  Md19Pos : Inport  Port=55
  Md19PosMax : Inport  Port=56
  Md19PosMin : Inport  Port=57
  Md20Pos : Inport  Port=58
  Md20PosMax : Inport  Port=59
  Md20PosMin : Inport  Port=60
  Md21Pos : Inport  Port=61
  Md21PosMax : Inport  Port=62
  Md21PosMin : Inport  Port=63
  Md22Pos : Inport  Port=64
  Md22PosMax : Inport  Port=65
  Md22PosMin : Inport  Port=66
  Md23Pos : Inport  Port=67
  Md23PosMax : Inport  Port=68
  Md23PosMin : Inport  Port=69
  Md24Pos : Inport  Port=70
  Md24PosMax : Inport  Port=71
  Md24PosMin : Inport  Port=72
  Md25Pos : Inport  Port=73
  Md25PosMax : Inport  Port=74
  Md25PosMin : Inport  Port=75
  Md26Pos : Inport  Port=76
  Md26PosMax : Inport  Port=77
  Md26PosMin : Inport  Port=78
  Md27Pos : Inport  Port=79
  Md27PosMax : Inport  Port=80
  Md27PosMin : Inport  Port=81
  Md28Pos : Inport  Port=82
  Md28PosMax : Inport  Port=83
  Md28PosMin : Inport  Port=84
  Md29Pos : Inport  Port=85
  Md29PosMax : Inport  Port=86
  Md29PosMin : Inport  Port=87
  Md30Pos : Inport  Port=88
  Md30PosMax : Inport  Port=89
  Md30PosMin : Inport  Port=90
  Md31Pos : Inport  Port=91
  Md31PosMax : Inport  Port=92
  Md31PosMin : Inport  Port=93
  Md32Pos : Inport  Port=94
  Md32PosMax : Inport  Port=95
  Md32PosMin : Inport  Port=96
  Mux : Mux  Inputs=32
  Mux{1..32} (32 alike) : Mux  Inputs=3
  CalibArray32 : Outport  VectorParamsAs1DForOutWhenUnconnected=off
  wires:
  Md22PosMax/1 -> Mux29/2
  Md3PosMin/1 -> Mux3/3
  Mux13/1 -> Mux/13
  Md13Pos/1 -> Mux13/1
  Mux30/1 -> Mux/23
  Md2PosMax/1 -> Mux2/2
  Md12PosMin/1 -> Mux12/3
  Md15PosMax/1 -> Mux15/2
  Md17Pos/1 -> Mux17/1
  Mux20/1 -> Mux/28
  Mux27/1 -> Mux/20
  Mux11/1 -> Mux/11
  Mux31/1 -> Mux/24
  Mux24/1 -> Mux/32
  Md8PosMin/1 -> Mux8/3
  Mux7/1 -> Mux/7
  Md20Pos/1 -> Mux27/1
  Mux6/1 -> Mux/6
  Md2PosMin/1 -> Mux2/3
  Md2Pos/1 -> Mux2/1
  Md5Pos/1 -> Mux5/1
  Md4PosMax/1 -> Mux4/2
  Mux25/1 -> Mux/18
  Md5PosMin/1 -> Mux5/3
  Md16PosMin/1 -> Mux16/3
  Md12PosMax/1 -> Mux12/2
  Mux32/1 -> Mux/25
  Md15PosMin/1 -> Mux15/3
  Mux15/1 -> Mux/15
  Mux16/1 -> Mux/16
  Mux21/1 -> Mux/29
  Md27PosMax/1 -> Mux19/2
  Md28Pos/1 -> Mux20/1
  Md13PosMin/1 -> Mux13/3
  Mux29/1 -> Mux/22
  Md8Pos/1 -> Mux8/1
  Mux23/1 -> Mux/31
  Mux22/1 -> Mux/30
  Mux12/1 -> Mux/12
  Md24Pos/1 -> Mux31/1
  Mux9/1 -> Mux/9
  Mux8/1 -> Mux/8
  Md9Pos/1 -> Mux9/1
  Mux3/1 -> Mux/3
  Md6PosMin/1 -> Mux6/3
  Mux17/1 -> Mux/17
  Md6Pos/1 -> Mux6/1
  Mux14/1 -> Mux/14
  Mux1/1 -> Mux/1
  Md10Pos/1 -> Mux10/1
  Md9PosMax/1 -> Mux9/2
  Mux26/1 -> Mux/19
  Mux18/1 -> Mux/26
  Mux28/1 -> Mux/21
  Mux2/1 -> Mux/2
  Mux19/1 -> Mux/27
  Mux10/1 -> Mux/10
  Mux5/1 -> Mux/5
  Md23PosMin/1 -> Mux30/3
  Md4PosMin/1 -> Mux4/3
  Md7PosMin/1 -> Mux7/3
  Md4Pos/1 -> Mux4/1
  Mux4/1 -> Mux/4
  Md13PosMax/1 -> Mux13/2
  Md6PosMax/1 -> Mux6/2
  Md5PosMax/1 -> Mux5/2
  Md14PosMax/1 -> Mux14/2
  Md14PosMin/1 -> Mux14/3
  Md23PosMax/1 -> Mux30/2
  Md1Min/1 -> Mux1/3
  Md8PosMax/1 -> Mux8/2
  Md23Pos/1 -> Mux30/1
  Md1Pos/1 -> Mux1/1
  Md1Max/1 -> Mux1/2
  Md9PosMin/1 -> Mux9/3
  Md7PosMax/1 -> Mux7/2
  Md20PosMin/1 -> Mux27/3
  Md7Pos/1 -> Mux7/1
  Md10PosMax/1 -> Mux10/2
  Md10PosMin/1 -> Mux10/3
  Md15Pos/1 -> Mux15/1
  Md30PosMax/1 -> Mux22/2
  Md11PosMax/1 -> Mux11/2
  Md12Pos/1 -> Mux12/1
  Md11PosMin/1 -> Mux11/3
  Md11Pos/1 -> Mux11/1
  Md14Pos/1 -> Mux14/1
  Md16Pos/1 -> Mux16/1
  Md24PosMin/1 -> Mux31/3
  Md16PosMax/1 -> Mux16/2
  Md32PosMin/1 -> Mux24/3
  Md27Pos/1 -> Mux19/1
  Md32PosMax/1 -> Mux24/2
  Md18Pos/1 -> Mux25/1
  Md19Pos/1 -> Mux26/1
  Md19PosMax/1 -> Mux26/2
  Md21Pos/1 -> Mux28/1
  Md27PosMin/1 -> Mux19/3
  Md26PosMax/1 -> Mux18/2
  Md26PosMin/1 -> Mux18/3
  Md31Pos/1 -> Mux23/1
  Md25Pos/1 -> Mux32/1
  Md28PosMin/1 -> Mux20/3
  Md25PosMin/1 -> Mux32/3
  Md25PosMax/1 -> Mux32/2
  Md17PosMin/1 -> Mux17/3
  Md32Pos/1 -> Mux24/1
  Md24PosMax/1 -> Mux31/2
  Md18PosMax/1 -> Mux25/2
  Md21PosMin/1 -> Mux28/3
  Md30PosMin/1 -> Mux22/3
  Md21PosMax/1 -> Mux28/2
  Md22Pos/1 -> Mux29/1
  Md18PosMin/1 -> Mux25/3
  Md26Pos/1 -> Mux18/1
  Md20PosMax/1 -> Mux27/2
  Md31PosMin/1 -> Mux23/3
  Md29Pos/1 -> Mux21/1
  Md19PosMin/1 -> Mux26/3
  Md29PosMin/1 -> Mux21/3
  Md30Pos/1 -> Mux22/1
  Md17PosMax/1 -> Mux17/2
  Md28PosMax/1 -> Mux20/2
  Md22PosMin/1 -> Mux29/3
  Md31PosMax/1 -> Mux23/2
  Md29PosMax/1 -> Mux21/2
  Mux/1 -> CalibArray32/1
  Md3Pos/1 -> Mux3/1
  Md3PosMax/1 -> Mux3/2

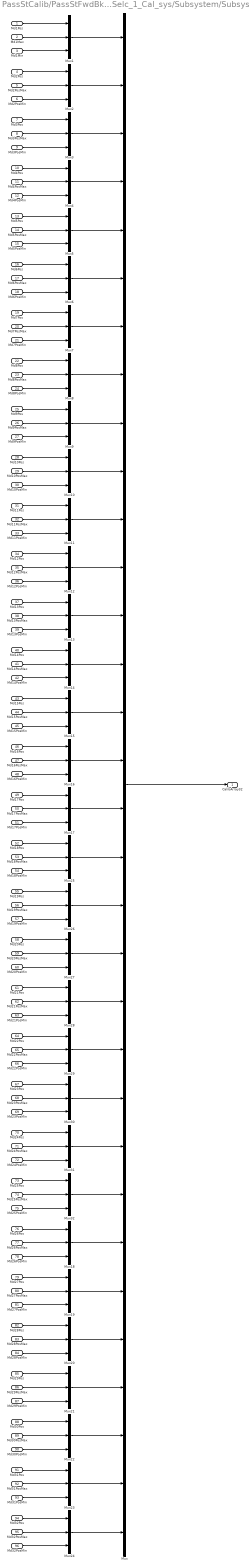
== system PassStCalib/PassStFwdBkwdTrgtPosSelc_1_Cal_sys/Subsystem/Subsystem ==
  Md1Pos : Inport
  Md1Max : Inport  Port=2
  Md1Min : Inport  Port=3
  Md2Pos : Inport  Port=4
  Md2PosMax : Inport  Port=5
  Md2PosMin : Inport  Port=6
  Md3Pos : Inport  Port=7
  Md3PosMax : Inport  Port=8
  Md3PosMin : Inport  Port=9
  Md4Pos : Inport  Port=10
  Md4PosMax : Inport  Port=11
  Md4PosMin : Inport  Port=12
  Md5Pos : Inport  Port=13
  Md5PosMax : Inport  Port=14
  Md5PosMin : Inport  Port=15
  Md6Pos : Inport  Port=16
  Md6PosMax : Inport  Port=17
  Md6PosMin : Inport  Port=18
  Md7Pos : Inport  Port=19
  Md7PosMax : Inport  Port=20
  Md7PosMin : Inport  Port=21
  Md8Pos : Inport  Port=22
  Md8PosMax : Inport  Port=23
  Md8PosMin : Inport  Port=24
  Md9Pos : Inport  Port=25
  Md9PosMax : Inport  Port=26
  Md9PosMin : Inport  Port=27
  Md10Pos : Inport  Port=28
  Md10PosMax : Inport  Port=29
  Md10PosMin : Inport  Port=30
  Md11Pos : Inport  Port=31
  Md11PosMax : Inport  Port=32
  Md11PosMin : Inport  Port=33
  Md12Pos : Inport  Port=34
  Md12PosMax : Inport  Port=35
  Md12PosMin : Inport  Port=36
  Md13Pos : Inport  Port=37
  Md13PosMax : Inport  Port=38
  Md13PosMin : Inport  Port=39
  Md14Pos : Inport  Port=40
  Md14PosMax : Inport  Port=41
  Md14PosMin : Inport  Port=42
  Md15Pos : Inport  Port=43
  Md15PosMax : Inport  Port=44
  Md15PosMin : Inport  Port=45
  Md16Pos : Inport  Port=46
  Md16PosMax : Inport  Port=47
  Md16PosMin : Inport  Port=48
  Md17Pos : Inport  Port=49
  Md17PosMax : Inport  Port=50
  Md17PosMin : Inport  Port=51
  Md18Pos : Inport  Port=52
  Md18PosMax : Inport  Port=53
  Md18PosMin : Inport  Port=54
  Md19Pos : Inport  Port=55
  Md19PosMax : Inport  Port=56
  Md19PosMin : Inport  Port=57
  Md20Pos : Inport  Port=58
  Md20PosMax : Inport  Port=59
  Md20PosMin : Inport  Port=60
  Md21Pos : Inport  Port=61
  Md21PosMax : Inport  Port=62
  Md21PosMin : Inport  Port=63
  Md22Pos : Inport  Port=64
  Md22PosMax : Inport  Port=65
  Md22PosMin : Inport  Port=66
  Md23Pos : Inport  Port=67
  Md23PosMax : Inport  Port=68
  Md23PosMin : Inport  Port=69
  Md24Pos : Inport  Port=70
  Md24PosMax : Inport  Port=71
  Md24PosMin : Inport  Port=72
  Md25Pos : Inport  Port=73
  Md25PosMax : Inport  Port=74
  Md25PosMin : Inport  Port=75
  Md26Pos : Inport  Port=76
  Md26PosMax : Inport  Port=77
  Md26PosMin : Inport  Port=78
  Md27Pos : Inport  Port=79
  Md27PosMax : Inport  Port=80
  Md27PosMin : Inport  Port=81
  Md28Pos : Inport  Port=82
  Md28PosMax : Inport  Port=83
  Md28PosMin : Inport  Port=84
  Md29Pos : Inport  Port=85
  Md29PosMax : Inport  Port=86
  Md29PosMin : Inport  Port=87
  Md30Pos : Inport  Port=88
  Md30PosMax : Inport  Port=89
  Md30PosMin : Inport  Port=90
  Md31Pos : Inport  Port=91
  Md31PosMax : Inport  Port=92
  Md31PosMin : Inport  Port=93
  Md32Pos : Inport  Port=94
  Md32PosMax : Inport  Port=95
  Md32PosMin : Inport  Port=96
  Mux : Mux  Inputs=32
  Mux{1..32} (32 alike) : Mux  Inputs=3
  CalibArray32 : Outport  VectorParamsAs1DForOutWhenUnconnected=off
  wires:
  Md22PosMax/1 -> Mux29/2
  Md3PosMin/1 -> Mux3/3
  Mux13/1 -> Mux/13
  Md13Pos/1 -> Mux13/1
  Mux30/1 -> Mux/23
  Md2PosMax/1 -> Mux2/2
  Md12PosMin/1 -> Mux12/3
  Md15PosMax/1 -> Mux15/2
  Md17Pos/1 -> Mux17/1
  Mux20/1 -> Mux/28
  Mux27/1 -> Mux/20
  Mux11/1 -> Mux/11
  Mux31/1 -> Mux/24
  Mux24/1 -> Mux/32
  Md8PosMin/1 -> Mux8/3
  Mux7/1 -> Mux/7
  Md20Pos/1 -> Mux27/1
  Mux6/1 -> Mux/6
  Md2PosMin/1 -> Mux2/3
  Md2Pos/1 -> Mux2/1
  Md5Pos/1 -> Mux5/1
  Md4PosMax/1 -> Mux4/2
  Mux25/1 -> Mux/18
  Md5PosMin/1 -> Mux5/3
  Md16PosMin/1 -> Mux16/3
  Md12PosMax/1 -> Mux12/2
  Mux32/1 -> Mux/25
  Md15PosMin/1 -> Mux15/3
  Mux15/1 -> Mux/15
  Mux16/1 -> Mux/16
  Mux21/1 -> Mux/29
  Md27PosMax/1 -> Mux19/2
  Md28Pos/1 -> Mux20/1
  Md13PosMin/1 -> Mux13/3
  Mux29/1 -> Mux/22
  Md8Pos/1 -> Mux8/1
  Mux23/1 -> Mux/31
  Mux22/1 -> Mux/30
  Mux12/1 -> Mux/12
  Md24Pos/1 -> Mux31/1
  Mux9/1 -> Mux/9
  Mux8/1 -> Mux/8
  Md9Pos/1 -> Mux9/1
  Mux3/1 -> Mux/3
  Md6PosMin/1 -> Mux6/3
  Mux17/1 -> Mux/17
  Md6Pos/1 -> Mux6/1
  Mux14/1 -> Mux/14
  Mux1/1 -> Mux/1
  Md10Pos/1 -> Mux10/1
  Md9PosMax/1 -> Mux9/2
  Mux26/1 -> Mux/19
  Mux18/1 -> Mux/26
  Mux28/1 -> Mux/21
  Mux2/1 -> Mux/2
  Mux19/1 -> Mux/27
  Mux10/1 -> Mux/10
  Mux5/1 -> Mux/5
  Md23PosMin/1 -> Mux30/3
  Md4PosMin/1 -> Mux4/3
  Md7PosMin/1 -> Mux7/3
  Md4Pos/1 -> Mux4/1
  Mux4/1 -> Mux/4
  Md13PosMax/1 -> Mux13/2
  Md6PosMax/1 -> Mux6/2
  Md5PosMax/1 -> Mux5/2
  Md14PosMax/1 -> Mux14/2
  Md14PosMin/1 -> Mux14/3
  Md23PosMax/1 -> Mux30/2
  Md1Min/1 -> Mux1/3
  Md8PosMax/1 -> Mux8/2
  Md23Pos/1 -> Mux30/1
  Md1Pos/1 -> Mux1/1
  Md1Max/1 -> Mux1/2
  Md9PosMin/1 -> Mux9/3
  Md7PosMax/1 -> Mux7/2
  Md20PosMin/1 -> Mux27/3
  Md7Pos/1 -> Mux7/1
  Md10PosMax/1 -> Mux10/2
  Md10PosMin/1 -> Mux10/3
  Md15Pos/1 -> Mux15/1
  Md30PosMax/1 -> Mux22/2
  Md11PosMax/1 -> Mux11/2
  Md12Pos/1 -> Mux12/1
  Md11PosMin/1 -> Mux11/3
  Md11Pos/1 -> Mux11/1
  Md14Pos/1 -> Mux14/1
  Md16Pos/1 -> Mux16/1
  Md24PosMin/1 -> Mux31/3
  Md16PosMax/1 -> Mux16/2
  Md32PosMin/1 -> Mux24/3
  Md27Pos/1 -> Mux19/1
  Md32PosMax/1 -> Mux24/2
  Md18Pos/1 -> Mux25/1
  Md19Pos/1 -> Mux26/1
  Md19PosMax/1 -> Mux26/2
  Md21Pos/1 -> Mux28/1
  Md27PosMin/1 -> Mux19/3
  Md26PosMax/1 -> Mux18/2
  Md26PosMin/1 -> Mux18/3
  Md31Pos/1 -> Mux23/1
  Md25Pos/1 -> Mux32/1
  Md28PosMin/1 -> Mux20/3
  Md25PosMin/1 -> Mux32/3
  Md25PosMax/1 -> Mux32/2
  Md17PosMin/1 -> Mux17/3
  Md32Pos/1 -> Mux24/1
  Md24PosMax/1 -> Mux31/2
  Md18PosMax/1 -> Mux25/2
  Md21PosMin/1 -> Mux28/3
  Md30PosMin/1 -> Mux22/3
  Md21PosMax/1 -> Mux28/2
  Md22Pos/1 -> Mux29/1
  Md18PosMin/1 -> Mux25/3
  Md26Pos/1 -> Mux18/1
  Md20PosMax/1 -> Mux27/2
  Md31PosMin/1 -> Mux23/3
  Md29Pos/1 -> Mux21/1
  Md19PosMin/1 -> Mux26/3
  Md29PosMin/1 -> Mux21/3
  Md30Pos/1 -> Mux22/1
  Md17PosMax/1 -> Mux17/2
  Md28PosMax/1 -> Mux20/2
  Md22PosMin/1 -> Mux29/3
  Md31PosMax/1 -> Mux23/2
  Md29PosMax/1 -> Mux21/2
  Mux/1 -> CalibArray32/1
  Md3Pos/1 -> Mux3/1
  Md3PosMax/1 -> Mux3/2
